simulink model "ColorBasedTracking"  (R2015b)
settings: Solver=ode45  StartTime=0.0  StopTime=30  RelTol=1e-3
values from neighbouring files (symbols this model uses):
  Kpa = 1    [ColorBasedTrackingCalc.m]
  Kpx = 0.1    [ColorBasedTrackingCalc.m]
  Kpy = 5    [ColorBasedTrackingCalc.m]
libraries: simulink x5
settings Model: Creator=zhang794  LastModifiedBy=aaeadmin
settings DataIOCC: SaveFormat=Array
settings HardwareCC: ProdBitPerPointer=32  ProdLargestAtomicFloat=None  ProdIntDivRoundTo=Undefined  ProdEndianess=Unspecified  ProdWordSize=32  ProdHWDeviceType=32-bit Generic
settings GRTTargetCC: GeneratePreprocessorConditionals=Disable all
settings ConfigComp: CovModelRefEnable=Off

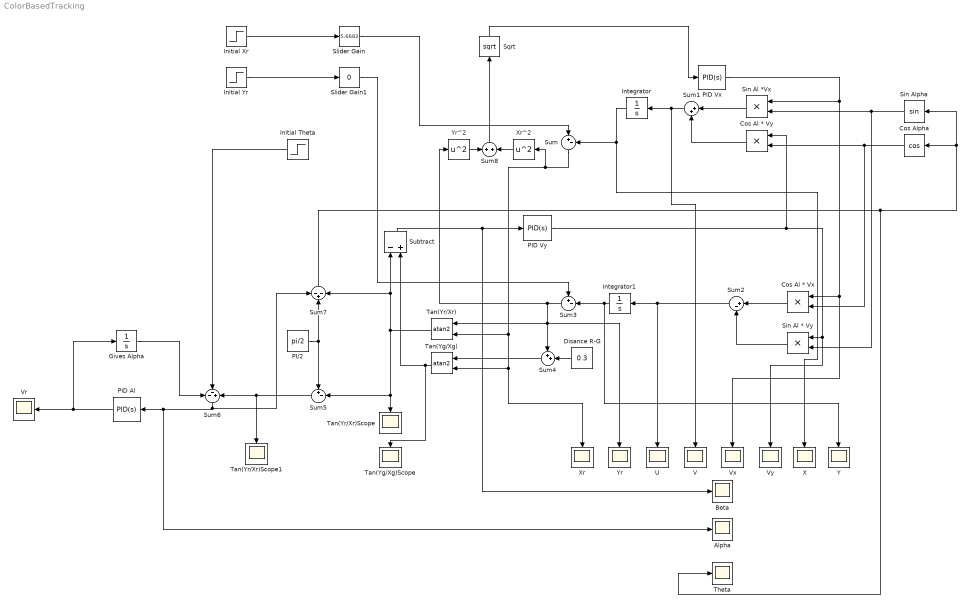
== system ColorBasedTracking ==
  Alpha : Scope
  Beta : Scope
  Cos Al * Vx : Product
  Cos Al * Vy : Product
  Cos Alpha : Trigonometry  Operator=cos  OutputSignalType=real
  Disance R-G : Constant  Value=0.3
  Gives Alpha : Integrator
  Initial Theta : Step  Time=0  After=0  SampleTime=0
  Initial Xr : Step  Time=0  SampleTime=0
  Initial Yr : Step  Time=0  SampleTime=0
  Integrator : Integrator
  Integrator1 : Integrator
  PI/2 : Constant  Value=pi/2
  PID Al : simulink/Continuous/PID Controller  Controller=PID  TimeDomain=Continuous-time  SampleTime=-1  IntegratorMethod=Forward Euler  FilterMethod=Forward Euler  Form=Parallel  UseFilter=on  ControllerParametersSource=internal  P=Kpa  I=0  D=0  N=100  InitialConditionSource=internal  InitialConditionForIntegrator=0  InitialConditionForFilter=0  ExternalReset=none  LimitOutput=off  UpperSaturationLimit=inf  LowerSaturationLimit=-inf  LinearizeAsGain=on  AntiWindupMode=none  Kb=1  TrackingMode=off  Kt=1  PParamMin=[]  PParamMax=[]  IParamMin=[]  IParamMax=[]  DParamMin=[]  DParamMax=[]  NParamMin=[]  NParamMax=[]  KbParamMin=[]  KbParamMax=[]  KtParamMin=[]  KtParamMax=[]  POutMin=[]  POutMax=[]  IOutMin=[]  IOutMax=[]  DOutMin=[]  DOutMax=[]  NOutMin=[]  NOutMax=[]  KbOutMin=[]  KbOutMax=[]  KtOutMin=[]  KtOutMax=[]  IntegratorOutMin=[]  IntegratorOutMax=[]  FilterOutMin=[]  FilterOutMax=[]  SumOutMin=[]  SumOutMax=[]  SumI1OutMin=[]  SumI1OutMax=[]  SumI2OutMin=[]  SumI2OutMax=[]  SumI3OutMin=[]  SumI3OutMax=[]  SumDOutMin=[]  SumDOutMax=[]  SaturationOutMin=[]  SaturationOutMax=[]  IntegratorContinuousStateAttributes=''  IntegratorStateMustResolveToSignalObject=off  IntegratorRTWStateStorageClass=Auto  FilterContinuousStateAttributes=''  FilterStateMustResolveToSignalObject=off  FilterRTWStateStorageClass=Auto  DifferentiatorICPrevScaledInput=0  DifferentiatorOutMin=[]  DifferentiatorOutMax=[]
  PID Vx : simulink/Continuous/PID Controller  Controller=PID  TimeDomain=Continuous-time  SampleTime=-1  IntegratorMethod=Forward Euler  FilterMethod=Forward Euler  Form=Parallel  UseFilter=on  ControllerParametersSource=internal  P=Kpx  I=0  D=0  N=100  InitialConditionSource=internal  InitialConditionForIntegrator=0  InitialConditionForFilter=0  ExternalReset=none  LimitOutput=off  UpperSaturationLimit=inf  LowerSaturationLimit=-inf  LinearizeAsGain=on  AntiWindupMode=none  Kb=1  TrackingMode=off  Kt=1  PParamMin=[]  PParamMax=[]  IParamMin=[]  IParamMax=[]  DParamMin=[]  DParamMax=[]  NParamMin=[]  NParamMax=[]  KbParamMin=[]  KbParamMax=[]  KtParamMin=[]  KtParamMax=[]  POutMin=[]  POutMax=[]  IOutMin=[]  IOutMax=[]  DOutMin=[]  DOutMax=[]  NOutMin=[]  NOutMax=[]  KbOutMin=[]  KbOutMax=[]  KtOutMin=[]  KtOutMax=[]  IntegratorOutMin=[]  IntegratorOutMax=[]  FilterOutMin=[]  FilterOutMax=[]  SumOutMin=[]  SumOutMax=[]  SumI1OutMin=[]  SumI1OutMax=[]  SumI2OutMin=[]  SumI2OutMax=[]  SumI3OutMin=[]  SumI3OutMax=[]  SumDOutMin=[]  SumDOutMax=[]  SaturationOutMin=[]  SaturationOutMax=[]  IntegratorContinuousStateAttributes=''  IntegratorStateMustResolveToSignalObject=off  IntegratorRTWStateStorageClass=Auto  FilterContinuousStateAttributes=''  FilterStateMustResolveToSignalObject=off  FilterRTWStateStorageClass=Auto  DifferentiatorICPrevScaledInput=0  DifferentiatorOutMin=[]  DifferentiatorOutMax=[]
  PID Vy : simulink/Continuous/PID Controller  Controller=PID  TimeDomain=Continuous-time  SampleTime=-1  IntegratorMethod=Forward Euler  FilterMethod=Forward Euler  Form=Parallel  UseFilter=on  ControllerParametersSource=internal  P=Kpy  I=0  D=0  N=100  InitialConditionSource=internal  InitialConditionForIntegrator=0  InitialConditionForFilter=0  ExternalReset=none  LimitOutput=off  UpperSaturationLimit=inf  LowerSaturationLimit=-inf  LinearizeAsGain=on  AntiWindupMode=none  Kb=1  TrackingMode=off  Kt=1  PParamMin=[]  PParamMax=[]  IParamMin=[]  IParamMax=[]  DParamMin=[]  DParamMax=[]  NParamMin=[]  NParamMax=[]  KbParamMin=[]  KbParamMax=[]  KtParamMin=[]  KtParamMax=[]  POutMin=[]  POutMax=[]  IOutMin=[]  IOutMax=[]  DOutMin=[]  DOutMax=[]  NOutMin=[]  NOutMax=[]  KbOutMin=[]  KbOutMax=[]  KtOutMin=[]  KtOutMax=[]  IntegratorOutMin=[]  IntegratorOutMax=[]  FilterOutMin=[]  FilterOutMax=[]  SumOutMin=[]  SumOutMax=[]  SumI1OutMin=[]  SumI1OutMax=[]  SumI2OutMin=[]  SumI2OutMax=[]  SumI3OutMin=[]  SumI3OutMax=[]  SumDOutMin=[]  SumDOutMax=[]  SaturationOutMin=[]  SaturationOutMax=[]  IntegratorContinuousStateAttributes=''  IntegratorStateMustResolveToSignalObject=off  IntegratorRTWStateStorageClass=Auto  FilterContinuousStateAttributes=''  FilterStateMustResolveToSignalObject=off  FilterRTWStateStorageClass=Auto  DifferentiatorICPrevScaledInput=0  DifferentiatorOutMin=[]  DifferentiatorOutMax=[]
  Sin Al * Vy : Product
  Sin Al *Vx : Product
  Sin Alpha : Trigonometry  OutputSignalType=real
  Slider Gain : simulink/Math Operations/Slider Gain  low=-10  gain=5.6682  high=10
  Slider Gain1 : simulink/Math Operations/Slider Gain  low=-10  gain=0  high=10
  Sqrt : Sqrt  SaturateOnIntegerOverflow=on
  Subtract : Sum  Inputs=-+
  Sum : Sum  Inputs=|+-
  Sum1 : Sum  Inputs=|++
  Sum2 : Sum  Inputs=|+-
  Sum3 : Sum  Inputs=+-|
  Sum4 : Sum  Inputs=++|
  Sum5 : Sum  Inputs=+-|
  Sum6 : Sum  Inputs=--+
  Sum7 : Sum  Inputs=-+-
  Sum8 : Sum  Inputs=+|+
  Tan(Yg/Xg) : Trigonometry  Operator=atan2  OutputSignalType=real
  Tan(Yg/Xg)Scope : Scope
  Tan(Yr/Xr) : Trigonometry  Operator=atan2  OutputSignalType=real
  Tan(Yr/Xr)Scope : Scope
  Tan(Yr/Xr)Scope1 : Scope
  "Theta " : Scope
  U : Scope
  V : Scope
  Vr : Scope
  Vx : Scope
  Vy : Scope
  X : Scope
  Xr : Scope
  Xr^2 : Math  Operator=square  SaturateOnIntegerOverflow=on
  Y : Scope
  Yr : Scope
  Yr^2 : Math  Operator=square  SaturateOnIntegerOverflow=on
  wires:
  Sum/1 -> Xr^2/1, Xr/1, Tan(Yg/Xg)/2, Tan(Yr/Xr)/2
  PID Vx/1 -> Cos Al * Vx/1, Vx/1, Sin Al *Vx/1
  Sin Al *Vx/1 -> Sum1/1
  Sum6/1 -> Sum7/1, PID Al/1, Alpha/1
  PID Vy/1 -> Vy/1, Sin Al * Vy/1, Cos Al * Vy/1
  Cos Al * Vy/1 -> Sum1/2
  Sum1/1 -> V/1, Integrator/1
  Integrator/1 -> X/1, Sum/2
  Cos Al * Vx/1 -> Sum2/1
  Sin Al * Vy/1 -> Sum2/2
  Sum2/1 -> Integrator1/1, U/1
  Integrator1/1 -> Sum3/2, Y/1
  Sum3/1 -> Yr^2/1, Sum4/1, Yr/1, Tan(Yr/Xr)/1
  Disance R-G/1 -> Sum4/2
  Sum4/1 -> Tan(Yg/Xg)/1
  Tan(Yg/Xg)/1 -> Tan(Yg/Xg)Scope/1, Subtract/2
  PID Al/1 -> Gives Alpha/1, Vr/1
  Initial Theta/1 -> Sum6/2
  Gives Alpha/1 -> Sum6/1
  Subtract/1 -> Beta/1, PID Vy/1
  Tan(Yr/Xr)/1 -> Sum7/3, Subtract/1, Tan(Yr/Xr)Scope/1, Sum5/2
  Sum5/1 -> Tan(Yr/Xr)Scope1/1, Sum6/3
  PI/2/1 -> Sum5/1, Sum7/2
  Sum7/1 -> Sin Alpha/1, Cos Alpha/1, "Theta "/1
  Sin Alpha/1 -> Sin Al * Vy/2, Sin Al *Vx/2
  Cos Alpha/1 -> Cos Al * Vx/2, Cos Al * Vy/2
  Xr^2/1 -> Sum8/2
  Yr^2/1 -> Sum8/1
  Sum8/1 -> Sqrt/1
  Sqrt/1 -> PID Vx/1
  Initial Xr/1 -> Slider Gain/1
  Slider Gain/1 -> Sum/1
  Slider Gain1/1 -> Sum3/1
  Initial Yr/1 -> Slider Gain1/1
